simulink model "V6NVektorModelWs"  (R2018b)
settings: Solver=ode45  StartTime=0.0  StopTime=50.0  MaxStep=0.1  RelTol=1e-3  EnableMultiTasking=on
model workspace (MAT data in the model file):
  F = [-1  0.5  0  0  0  0  0  0  0  0  0  0  0  0  0; 0.5  -1  0.5  0  0  0  0  0  0  0  0  0  0  0  0; 0  0.5  -1  0.5  0  0  0  0  0  0  0  0  0  0  0; 0  0  0.5  -1  0.5  0  0  0  0  0  0  0  0  0  0; 0  0  0  0.5  -1  0.5  0  0  0  0  0  0  0  0  0; 0  0  0  0  0.5  -1  0.5  0  0  0  0  0  0  0  0; 0  0  0  0  0  0.5  -1  0.5  0  0  0  0  0  0  0; 0  0  0  0  0  0  0.5  -1  0.5  0  0  0  0  0  0; 0  0  0  0  0  0  0  0.5  -1  0.5  0  0  0  0  0; 0  0  0  0  0  0  0  0  0.5  -1  0.5  0  0  0  0; 0  0  0  0  0  0  0  0  0  0.5  -1  0.5  0  0  0; 0  0  0  0  0  0  0  0  0  0  0.5  -1  0.5  0  0; 0  0  0  0  0  0  0  0  0  0  0  0.5  -1  0.5  0; 0  0  0  0  0  0  0  0  0  0  0  0  0.5  -1  0.5; 0  0  0  0  0  0  0  0  0  0  0  0  0  0.5  -1]
  N = 15
  v0 = [0; 0; 0; 0; 0; 0; 0; 0; 0; 0; 0; 0; 0; 0; 0]
  x0 = [1; 0; 1; 1; 1; 1; 1; 1; 1; 1; 1; 1; 1; 1; 1]
settings Model: Creator=Reichl  LastModifiedBy=Reichl
settings DataIOCC: SaveFormat=Array  SignalLoggingSaveFormat=ModelDataLogs
settings OptimizationCC: ExpressionDepthLimit=2147483647  LifeSpan=inf
settings DebuggingCC: UnderspecifiedInitializationDetection=Classic  MergeDetectMultiDrivingBlocksExec=none  SolverPrmCheckMsg=warning  FcnCallInpInsideContextMsg=warning  AllowSymbolicDim=off  StateNameClashWarn=warning  SFUnexpectedBacktrackingDiag=warning  SFNoUnconditionalDefaultTransitionDiag=warning  SFExecutionAtInitializationDiag=none
settings HardwareCC: ProdBitPerPointer=32  ProdBitPerSizeT=32  ProdBitPerPtrDiffT=32  ProdLargestAtomicFloat=None  ProdIntDivRoundTo=Undefined  ProdEndianess=Unspecified  ProdWordSize=32  ProdHWDeviceType=32-bit Generic
settings ModelReferenceCC: PropagateSignalLabelsOutOfModel=off
settings SFSimCC: SimUseLocalCustomCode=off
settings RTWCC: RTWUseLocalCustomCode=off
settings CodeAppCC: StateflowObjectComments=on
settings GRTTargetCC: TargetLangStandard=C89/C90 (ANSI)  GeneratePreprocessorConditionals=Disable all  CombineOutputUpdateFcns=off  GRTInterface=on
settings ConfigComp: CovMetricSettings=dw  CovHtmlReporting=on  CovSaveCumulativeToWorkspaceVar=on  CovSaveSingleToWorkspaceVar=on  CovExternalEMLEnable=off  CovSFcnEnable=off

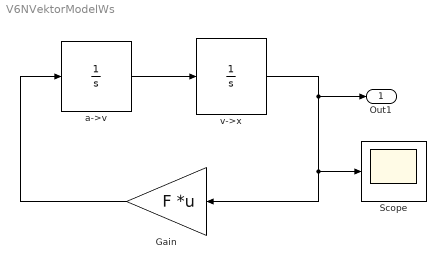
== system V6NVektorModelWs ==
  Gain : Gain  Gain=F  Multiplication=Matrix(K*u)
  Scope : Scope
  a->v : Integrator  InitialCondition=v0
  v->x : Integrator  InitialCondition=x0
  Out1 : Outport
  wires:
  a->v/1 -> v->x/1
  v->x/1 -> Gain/1, Scope/1, Out1/1
  Gain/1 -> a->v/1
